simulink model "mpcSetpointQuadprogNoOffset"  (Simulink 7.9)
settings: Solver=ode4  StartTime=0.0  StopTime=200  RelTol=1e-3
values from neighbouring files (symbols this model uses):
  A = params.A    [cvxsolve.m]    (also in prepSoftFewerSlacks.m = [1 dt 0.5*dt*dt; prepSoftKS.m = [1 dt 0.5*dt*dt; prepSoftKS_coupled.m = [1 dt 0.5*dt*dt; prepSoftQuadprog.m = [1 dt 0.5*dt*dt)
  b = [zeros(T*n,1); ef]    [prepSoftFewerSlacks.m]    (also in prepSoftKS.m; prepSoftKS_coupled.m; prepSoftQuadprog.m)
  B = params.B    [cvxsolve.m]    (also in prepSoftFewerSlacks.m = B*[1 0]; prepSoftKS.m = [0.5*dt*dt; prepSoftKS_coupled.m = [0.5*dt*dt; prepSoftQuadprog.m = B*[1 0])
  bd = [kron(ones(T,1),eye(n)); zeros(ellef,n)]    [prepSoftFewerSlacks.m]    (also in prepSoftKS.m = [kron(ones(T,1),eye(n)); [1 0 0; 0 1 0]]; prepSoftKS_coupled.m = [kron(ones(T,1),eye(n)); [1 0 0; 0 1 0]]; prepSoftQuadprog.m = [kron(ones(T,1),eye(n))])
  bx = [A; zeros(ellef+(T-1)*n,n)]    [prepSoftFewerSlacks.m]    (also in prepSoftKS.m; prepSoftKS_coupled.m; prepSoftQuadprog.m)
  C = [kron(eye(T),[-B eye(n)]) + kron([zeros(1,T); eye(T-1) zeros(T-1,1)],[zeros(n,m) -A]); zeros(ellef,m+(T-1)*(m+n)) Ef]    [prepSoftFewerSlacks.m]    (also in prepSoftKS.m; prepSoftKS_coupled.m; prepSoftQuadprog.m)
  dt = 0.25    [prepSoftFewerSlacks.m]    (also in prepSoftKS.m; prepSoftKS_coupled.m; prepSoftQuadprog.m)
  g = [r; repmat([q;r],T-1,1); qf]    [prepSoftFewerSlacks.m]    (also in prepSoftKS.m; prepSoftKS_coupled.m; prepSoftQuadprog.m)
  gt = kron(ones(T,1),[zeros(2,n); -2*Q])    [prepSoftFewerSlacks.m]    (also in prepSoftKS.m = kron(ones(T,1),[zeros(1,n); -2*Q]); prepSoftKS_coupled.m = kron(ones(T,1),[zeros(1,n); -2*Q]); prepSoftQuadprog.m)
  H = blkdiag(R,kron(eye(T-1),blkdiag(Q,R)),Qf)    [prepSoftFewerSlacks.m]    (also in prepSoftKS.m; prepSoftKS_coupled.m; prepSoftQuadprog.m)
  hc = [repmat(f,T,1);ff]    [prepSoftFewerSlacks.m]    (also in prepSoftKS.m; prepSoftKS_coupled.m; prepSoftQuadprog.m)
  hx = [-Fx; zeros((T-1)*ell + ellf,n)]    [prepSoftFewerSlacks.m]    (also in prepSoftKS.m; prepSoftKS_coupled.m; prepSoftQuadprog.m)
  m = size(B,2)    [ipoptSolve.m]    (also in ipoptSolve2.m; mpcsolve.m; mpcsolve_ipopt.m; prepSoftFewerSlacks.m)
  n = size(A,1)    [ipoptSolve.m]    (also in ipoptSolve2.m; mpcsolve.m = size(AT,1)/2; mpcsolve_ipopt.m; prepSoftFewerSlacks.m)
  P = blkdiag(Fu,kron(eye(T-1),[Fx Fu]),Ff)    [prepSoftFewerSlacks.m]    (also in prepSoftKS.m; prepSoftKS_coupled.m; prepSoftQuadprog.m)
  T = linsolve(cholM,eye(size(M,1)),struct('LT',true))    [ipoptSolve.m]    (also in ipoptSolve2.m; mpcsolve.m = (ne-ellef)/size(A,1); mpcsolve_ipopt.m; prepSoftFewerSlacks.m = 10)
undefined symbols (not defined in the file or in its folder): quadprog
libraries: simulink x1
settings Model: Creator=aeagr  LastModifiedBy=aeagr
settings DebuggingCC: FcnCallInpInsideContextMsg=Use local settings  StrictBusMsg=Warning
settings GRTTargetCC: CombineOutputUpdateFcns=off  GRTInterface=on

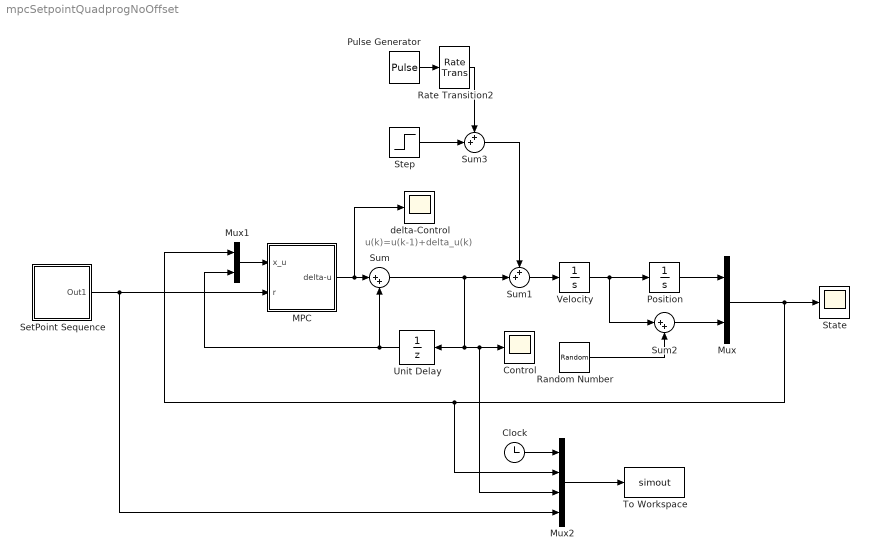
== system mpcSetpointQuadprogNoOffset ==
  note: u(k)=u(k-1)+delta_u(k)
  Clock : Clock
  Control : Scope
      settings: TimeRange=240  YMin=-0.4  YMax=0.35
  MPC : Subsystem  TreatAsAtomicUnit=on  SystemSampleTime=dt
  Mux : Mux  Inputs=2
  Mux1 : Mux  Inputs=2
  Mux2 : Mux
  Position : Integrator
  Pulse Generator : DiscretePulseGenerator  PulseType=Time based  Amplitude=-0.2*0  Period=200  PhaseDelay=120
  Random Number : RandomNumber  Variance=0.000000001  SampleTime=dt
  Rate Transition2 : RateTransition
  SetPoint Sequence : Subsystem
  State : Scope
      settings: TimeRange=200  YMin=-0.3  YMax=1
  Step : Step  Time=100  After=0.01  SampleTime=0
  Sum : Sum  Inputs=|++
  Sum1 : Sum  Inputs=++|
  Sum2 : Sum  Inputs=|++
  Sum3 : Sum  Inputs=++|
  To Workspace : ToWorkspace  VariableName=simout  SampleTime=-1
  Unit Delay : UnitDelay  SampleTime=dt
  Velocity : Integrator
  delta-Control : Scope
      settings: TimeRange=240  YMin=-0.4  YMax=0.35  SaveName=ScopeData2
  wires:
  Velocity/1 -> Position/1, Sum2/1
  Mux/1 -> State/1, Mux2/2, Mux1/1
  Position/1 -> Mux/1
  SetPoint Sequence/1(Out1) -> Mux2/4, MPC/2(r)
  Sum/1 -> Unit Delay/1, Control/1, Mux2/3, Sum1/2
  Unit Delay/1 -> Sum/2, Mux1/2
  MPC/1(delta-u) -> Sum/1, delta-Control/1
  Mux1/1 -> MPC/1(x_u)
  Sum1/1 -> Velocity/1
  Mux2/1 -> To Workspace/1
  Clock/1 -> Mux2/1
  Step/1 -> Sum3/2
  Pulse Generator/1 -> Rate Transition2/1
  Rate Transition2/1 -> Sum3/1
  Sum3/1 -> Sum1/1
  Sum2/1 -> Mux/2
  Random Number/1 -> Sum2/2

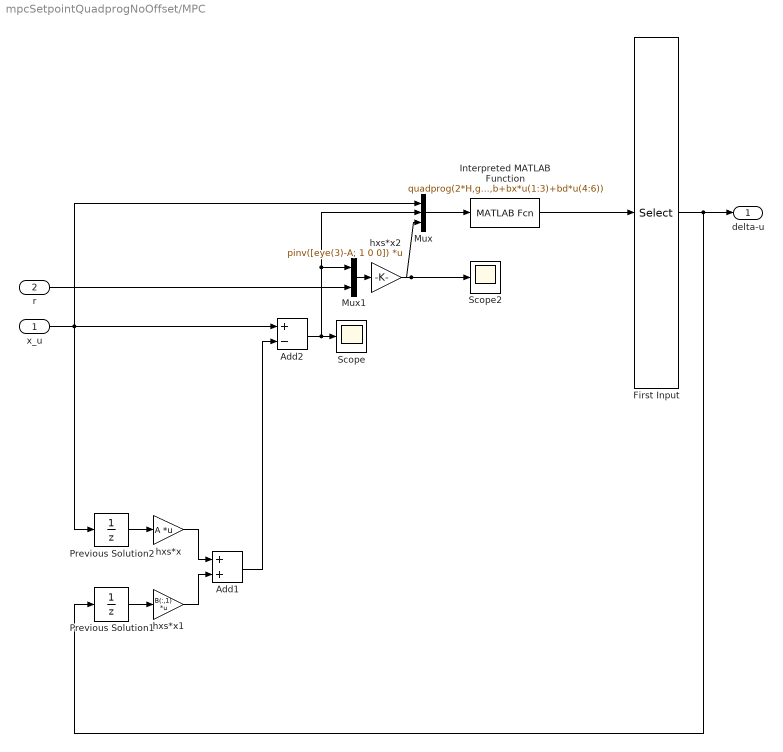
== system mpcSetpointQuadprogNoOffset/MPC ==
  x_u : Inport
  r : Inport  Port=2
  Add1 : Sum
  Add2 : Sum  Inputs=+-
  First Input : Selector  InputPortWidth=T*(n+m)  IndexOptions=Index vector (dialog)  Indices=1  OutputSizes=1
  Interpreted MATLAB Function : MATLABFcn  MATLABFcn=quadprog(2*H,g+gt*u(7:9),P,hx*u(1:3)+hc,C,b+bx*u(1:3)+bd*u(4:6))
  Mux : Mux  Inputs=3
  Mux1 : Mux  Inputs=2
  Previous Solution1 : UnitDelay  SampleTime=-1
  Previous Solution2 : UnitDelay  X0=[0 0 0]  SampleTime=-1
  Scope : Scope
      settings: YMin=0  YMax=0.00275  SaveName=ScopeData3
  Scope2 : Scope
      settings: YMin=0  YMax=0.00275  SaveName=ScopeData5
  hxs*x : Gain  Gain=A  Multiplication=Matrix(K*u)
  hxs*x1 : Gain  Gain=B(:,1)  Multiplication=Matrix(K*u)
  hxs*x2 : Gain  Gain=pinv([eye(3)-A; 1 0 0])  Multiplication=Matrix(K*u)
  delta-u : Outport
  wires:
  First Input/1 -> delta-u/1, Previous Solution1/1
  Interpreted MATLAB Function/1 -> First Input/1
  x_u/1 -> Previous Solution2/1, Add2/1, Mux/1
  hxs*x/1 -> Add1/1
  Previous Solution1/1 -> hxs*x1/1
  Add1/1 -> Add2/2
  Previous Solution2/1 -> hxs*x/1
  hxs*x1/1 -> Add1/2
  Mux/1 -> Interpreted MATLAB Function/1
  Add2/1 -> Scope/1, Mux/2, Mux1/1
  r/1 -> Mux1/2
  Mux1/1 -> hxs*x2/1
  hxs*x2/1 -> Scope2/1, Mux/3

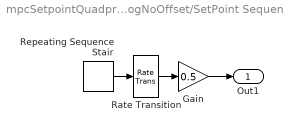
== system mpcSetpointQuadprogNoOffset/SetPoint Sequence ==
  Gain : Gain  Gain=0.5
  Rate Transition : RateTransition
  Repeating Sequence Stair : simulink/Sources/Repeating Sequence Stair  OutValues=[1 0 2 0 3 0 4 0 5 0 6 0].'  tsamp=20  OutMin=[]  OutMax=[]  OutDataTypeStr=double  OutputDataTypeScalingMode=Specify via dialog  OutDataType=double  ConRadixGroup=Best Precision: Vector-wise  OutScaling=2^-12
  Out1 : Outport
  wires:
  Repeating Sequence Stair/1 -> Rate Transition/1
  Rate Transition/1 -> Gain/1
  Gain/1 -> Out1/1
